simulink library "ESTS_LSM_DEC"  (R2023b)
settings: Solver=VariableStepAuto  StartTime=0.0  StopTime=10.0  RelTol=1e-3
undefined symbols (not defined in the file or in its folder): ESTS_LSM_DEC_p_SpdLgtMdlThd_kmph
libraries: VUT_lib x1
settings Model: Creator=blatak  LastModifiedBy=blatak

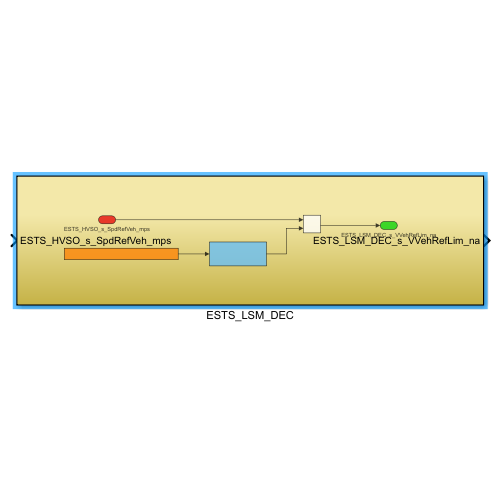
[thumbnail: Simulink's stored preview of the top-level diagram]
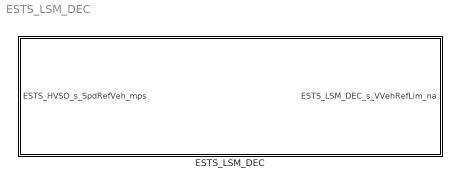
== system ESTS_LSM_DEC ==
  ESTS_LSM_DEC : Subsystem

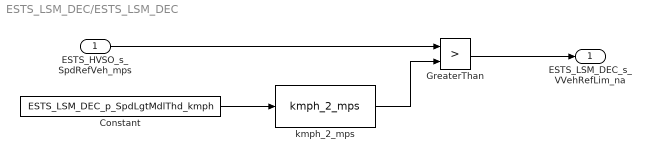
== system ESTS_LSM_DEC/ESTS_LSM_DEC ==
  ESTS_HVSO_s_SpdRefVeh_mps : Inport  Description=ESTS_HVSO_s_SpdRefVeh_mps
  Constant : Constant  Description=Parameter - limit of speed to switch between single track models  Value=ESTS_LSM_DEC_p_SpdLgtMdlThd_kmph
  GreaterThan : RelationalOperator  Operator=>  OutDataTypeStr=boolean  RndMeth=Simplest  InputSameDT=off
  kmph_2_mps : VUT_lib/kmph_2_mps  SystemSampleTime=-1  VariantActivationTime=update diagram  AllowFlexibleInterface=on  Latency=0  AutoFrameSizeCalculation=off
  ESTS_LSM_DEC_s_VVehRefLim_na : Outport  Description=Determination if the threshold velocity is reached, for switch use
  wires:
  GreaterThan/1 -> ESTS_LSM_DEC_s_VVehRefLim_na/1
  Constant/1 -> kmph_2_mps/1
  ESTS_HVSO_s_SpdRefVeh_mps/1 -> GreaterThan/1
  kmph_2_mps/1 -> GreaterThan/2
